simulink model "simulinknorm1"  (R2020b)
settings: Solver=VariableStepAuto  StartTime=0.0  StopTime=10.0  RelTol=1e-3
values from neighbouring files (symbols this model uses):
  A = [0 0 1 0 0;0 -0.154 -0.0042 1.54 0;0 0.249 -1 -5.2 0 ... (first row only)    [ac3mpccontroller.m]    (also in plantac3.m)
  B = [0 0;-0.744 -0.032;0.337 -1.12;0.02 0;0 0]    [ac3mpccontroller.m]    (also in plantac3.m)
  C = [0 1  0 0 -1;0 0 1 0 0;0 0 0 1 0;1 0 0 0 0]    [ac3mpccontroller.m]    (also in plantac3.m)
  nu = 2    [ac3mpccontroller.m]    (also in plantac3.m)
  nx = 5    [ac3mpccontroller.m]    (also in plantac3.m)
  ny = 4    [ac3mpccontroller.m]    (also in plantac3.m)
  Ts = .1    (= 0.1)    [ac3mpccontroller.m]    (also in plantac3.m)
  x0 = ones(nx,1)    [plantac3.m]
undefined symbols (not defined in the file or in its folder): ac3mpccontroller, DiscIntNeverNeededParam
libraries: simulink x2, dspmtrx3 x2
settings Model: Creator=shima  LastModifiedBy=shima

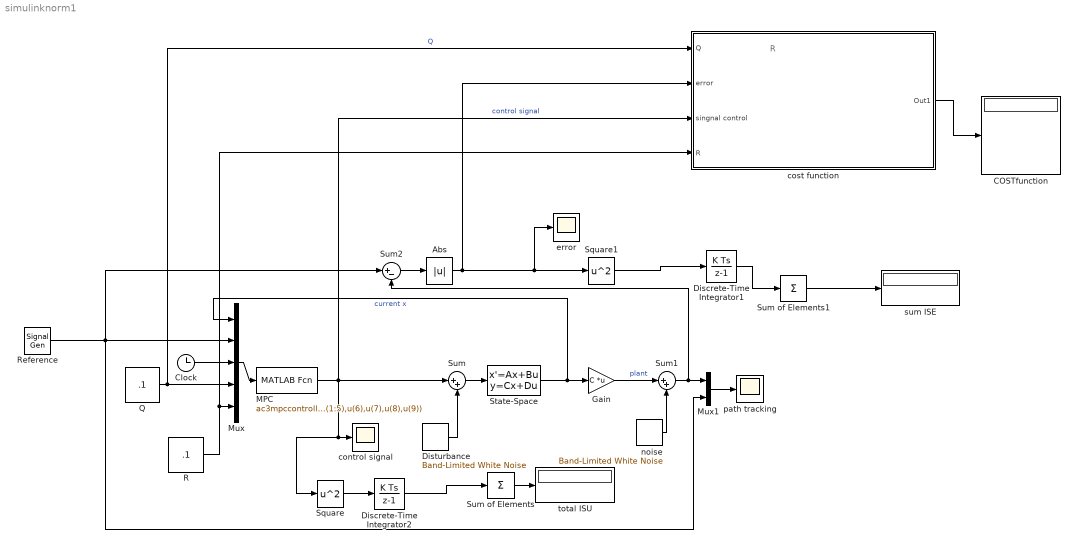
== system simulinknorm1 ==
  note: R
  Abs : Abs
  COSTfunction : Display
  Clock : Clock
  Discrete-Time Integrator1 : DiscreteIntegrator  SampleTime=-1  ICPrevOutput=DiscIntNeverNeededParam  ICPrevScaledInput=DiscIntNeverNeededParam
  Discrete-Time Integrator2 : DiscreteIntegrator  SampleTime=-1  ICPrevOutput=DiscIntNeverNeededParam  ICPrevScaledInput=DiscIntNeverNeededParam
  Disturbance : simulink/Sources/Band-Limited White Noise  Cov=[.01 .01]  Ts=0.1  seed=[23341]
  Gain : Gain  Gain=C  Multiplication=Matrix(K*u)
  MPC : MATLABFcn  Description=MPC controller  MATLABFcn=ac3mpccontroller(u(1:5),u(6),u(7),u(8),u(9))  SampleTime=Ts
  Mux : Mux  Inputs=5
  Mux1 : Mux  Inputs=2
  Q : Constant  Value=.1  SampleTime=-1
  R : Constant  Value=.1  SampleTime=-1
  Reference : SignalGenerator  WaveForm=square  Frequency=.2
  Square : Math  Operator=square  SaturateOnIntegerOverflow=on
  Square1 : Math  Operator=square  SaturateOnIntegerOverflow=on
  State-Space : StateSpace  A=A  B=B  C=eye(nx)  D=zeros(nx,nu)  InitialCondition=x0
  Sum : Sum  Inputs=|++
  Sum of Elements : Sum  Inputs=+
  Sum of Elements1 : Sum  Inputs=+
  Sum1 : Sum  Inputs=|++
  Sum2 : Sum  Inputs=|+-
  control signal : Scope
  cost function : Subsystem
  error : Scope
  noise : simulink/Sources/Band-Limited White Noise  Cov=[.001 .001 .01 .001]  Ts=0.1  seed=[23341]
  path tracking : Scope
  sum ISE : Display
  total ISU : Display
  wires:
  Sum2/1 -> Abs/1
  Sum of Elements/1 -> total ISU/1
  Discrete-Time Integrator1/1 -> Sum of Elements1/1
  Sum1/1 -> Sum2/2, Mux1/1
  cost function/1(Out1) -> COSTfunction/1
  noise/1 -> Sum1/2
  Square1/1 -> Discrete-Time Integrator1/1
  Sum of Elements1/1 -> sum ISE/1
  Discrete-Time Integrator2/1 -> Sum of Elements/1
  Mux1/1 -> path tracking/1
  Abs/1 -> cost function/2(error), error/1, Square1/1
  Disturbance/1 -> Sum/2
  Clock/1 -> Mux/3
  R/1 -> cost function/4(R), Mux/5
  Reference/1 -> Mux/2, Sum2/1, Mux1/2
  Mux/1 -> MPC/1
  MPC/1 -> Square/1, control signal/1, cost function/3(singnal control), Sum/1  "control signal"
  State-Space/1 -> Gain/1, Mux/1  "current x"
  Gain/1 -> Sum1/1  "plant"
  Sum/1 -> State-Space/1
  Square/1 -> Discrete-Time Integrator2/1
  Q/1 -> Mux/4, cost function/1(Q)  "Q"

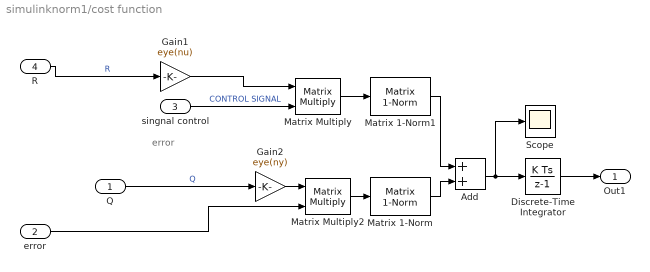
== system simulinknorm1/cost function ==
  note: error
  Q : Inport
  error : Inport  Port=2
  singnal control : Inport  Port=3
  R : Inport  Port=4
  Add : Sum
  Discrete-Time Integrator : DiscreteIntegrator  SampleTime=-1  ICPrevOutput=DiscIntNeverNeededParam  ICPrevScaledInput=DiscIntNeverNeededParam
  Gain1 : Gain  Gain=eye(nu)
  Gain2 : Gain  Gain=eye(ny)
  Matrix 1-Norm : dspmtrx3/Matrix  1-Norm  roundingMode=Floor  overflowMode=off  outputDataTypeStr=Inherit: Same as accumulator  outputMin=[]  outputMax=[]  outputLastDataTypeStr=Inherit: Same as accumulator
      settings: SourceProductBaseCode=DS
  Matrix 1-Norm1 : dspmtrx3/Matrix  1-Norm  roundingMode=Floor  overflowMode=off  outputDataTypeStr=Inherit: Same as accumulator  outputMin=[]  outputMax=[]  outputLastDataTypeStr=Inherit: Same as accumulator
      settings: SourceProductBaseCode=DS
  Matrix Multiply : Product  Multiplication=Matrix(*)
  Matrix Multiply2 : Product  Multiplication=Matrix(*)
  Scope : Scope
  Out1 : Outport
  wires:
  R/1 -> Gain1/1  "R"
  Q/1 -> Gain2/1  "Q"
  Add/1 -> Scope/1, Discrete-Time Integrator/1
  Discrete-Time Integrator/1 -> Out1/1
  error/1 -> Matrix Multiply2/2
  Gain2/1 -> Matrix Multiply2/1
  Matrix Multiply2/1 -> Matrix 1-Norm/1
  Matrix 1-Norm/1 -> Add/2
  Gain1/1 -> Matrix Multiply/1
  singnal control/1 -> Matrix Multiply/2  "CONTROL SIGNAL"
  Matrix Multiply/1 -> Matrix 1-Norm1/1
  Matrix 1-Norm1/1 -> Add/1
